simulink model "kinematic_arm_simulation"  (Simulink 7.8)
settings: Solver=FixedStepDiscrete  SolverMode=SingleTasking  StartTime=0.0  StopTime=50  FixedStep=.01  RelTol=1e-3  AbsTol=1e-6
undefined symbols (not defined in the file or in its folder): DiscIntNeverNeededParam, forward_kinematics, inverse_kinematics
libraries: simulink x2
settings Model: Creator=sschaal  LastModifiedBy=okhan  ExtModeAutoUpdateStatusClock=off
settings DataIOCC: LimitDataPoints=off  SaveOutput=off
settings OptimizationCC: BlockReduction=off  BooleanDataType=off  InitFltsAndDblsToZero=on
settings DebuggingCC: SaveWithParameterizedLinksMsg=none  SignalResolutionControl=TryResolveAllWithWarning  SolverPrmCheckMsg=none  MultiTaskDSMMsg=warning  MultiTaskCondExecSysMsg=none  FcnCallInpInsideContextMsg=Use local settings  StrictBusMsg=None
settings HardwareCC: TargetUnknown=on
settings RTWCC: IncludeERTFirstTime=on
settings GRTTargetCC: TargetFcnLib=ansi_tfl_tmw.mat

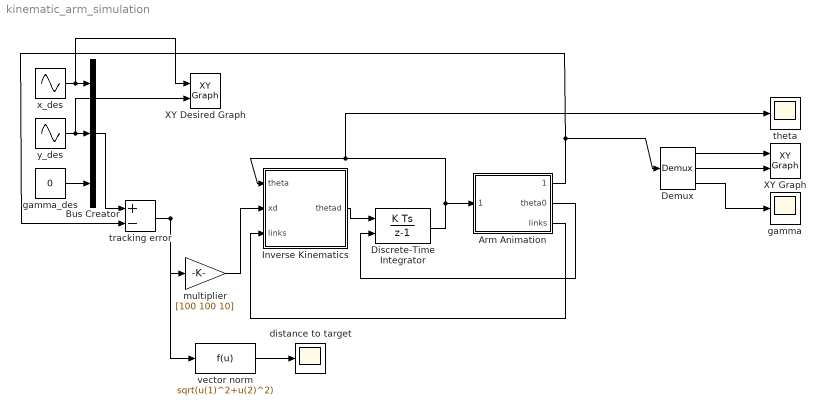
== system kinematic_arm_simulation ==
  Arm Animation : Subsystem  mask(ArmAnimation){links=[0.1 0.0 0.1 0.0 0.1 0.0 0.1 0.0], theta0=[0.0; 0.125; 0.0; 0.125; 0.0; 0.125; 0.0; 0.125], ts=.05}
      mask prompts: links "Link Lengths"; theta0 "Initial Posture"; ts "Sample time:"
  Bus Creator : BusCreator  Inputs=3
  Demux : Demux  Outputs=3
  Discrete-Time Integrator : DiscreteIntegrator  InitialConditionSource=external  SampleTime=0.01  UpperSaturationLimit=[inf .1 inf .1 inf .1 inf .1]  LowerSaturationLimit=[-inf 0 -inf 0 -inf 0 -inf 0]  ICPrevOutput=DiscIntNeverNeededParam  ICPrevScaledInput=DiscIntNeverNeededParam
  Inverse Kinematics : Subsystem
      mask Type: Inverse Kinematics
  XY Desired Graph : simulink/Sinks/XY Graph  xmin=0.2  xmax=1  ymin=-1  ymax=1  st=-1
  XY Graph : simulink/Sinks/XY Graph  xmin=0.2  xmax=1  ymin=-1  ymax=1  st=-1
  distance to target : Scope
      settings: TickLabels=on  TimeRange=50  YMin=0  YMax=0.016  DataFormat=Array
  gamma : Scope
      settings: TimeRange=50  YMin=-3e-15  YMax=5e-15
  gamma_des : Constant  Value=0
  multiplier : Gain  Gain=[100 100 10]  SaturateOnIntegerOverflow=on  OutDataTypeStr=Inherit: Same as input  ParamDataTypeStr=Inherit: Same as input
  theta : Scope
      settings: YMin=-0.8  YMax=0.9  SaveName=ScopeData2
  tracking error : Sum  Inputs=+-  SaturateOnIntegerOverflow=on  InputSameDT=on  OutDataTypeStr=Inherit: Same as first input
  vector norm : Fcn  Expr=sqrt(u(1)^2+u(2)^2)
  x_des : Sin  Amplitude=.3  Bias=.6  Frequency=pi/5  Phase=pi/2  SampleTime=0
  y_des : Sin  Amplitude=.6  Frequency=pi/5  SampleTime=0
  wires:
  multiplier/1 -> Inverse Kinematics/2(xd)
  Inverse Kinematics/1(thetad) -> Discrete-Time Integrator/1
  Discrete-Time Integrator/1 -> Arm Animation/1(Position), Inverse Kinematics/1(theta), theta/1
  Demux/1 -> XY Graph/1
  Demux/2 -> XY Graph/2
  Arm Animation/3(links) -> Inverse Kinematics/3(links)
  Arm Animation/2(theta0) -> Discrete-Time Integrator/2
  Arm Animation/1("[x,y,gamma]") -> tracking error/2, Demux/1
  tracking error/1 -> multiplier/1, vector norm/1
  vector norm/1 -> distance to target/1
  Bus Creator/1 -> tracking error/1
  x_des/1 -> Bus Creator/1, XY Desired Graph/1
  y_des/1 -> Bus Creator/2, XY Desired Graph/2
  gamma_des/1 -> Bus Creator/3
  Demux/3 -> gamma/1

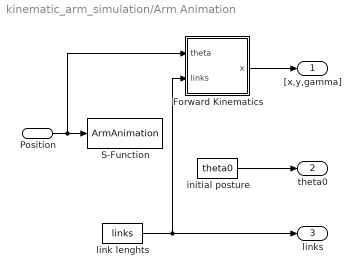
== system kinematic_arm_simulation/Arm Animation ==
  Position : Inport
  Forward Kinematics : Subsystem
      mask Type: Forward Kinematics
  S-Function : S-Function  FunctionName=ArmAnimation  Parameters=ts,theta0,links  EnableBusSupport=off
  initial posture : Constant  Value=theta0
  link lenghts : Constant  Value=links
  "[x,y,gamma]" : Outport
  theta0 : Outport  Port=2
  links : Outport  Port=3
  wires:
  initial posture/1 -> theta0/1
  Position/1 -> S-Function/1, Forward Kinematics/1(theta)
  Forward Kinematics/1(x) -> "[x,y,gamma]"/1
  link lenghts/1 -> links/1, Forward Kinematics/2(links)

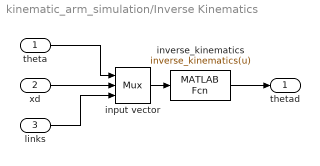
== system kinematic_arm_simulation/Inverse Kinematics ==
  theta : Inport
  xd : Inport  Port=2
  links : Inport  Port=3
  input vector : Mux  Inputs=3
  inverse_kinematics : MATLABFcn  MATLABFcn=inverse_kinematics(u)  OutputDimensions=8
  thetad : Outport  InitialOutput=0
  wires:
  theta/1 -> input vector/1
  xd/1 -> input vector/2
  input vector/1 -> inverse_kinematics/1
  links/1 -> input vector/3
  inverse_kinematics/1 -> thetad/1

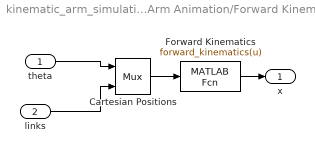
== system kinematic_arm_simulation/Arm Animation/Forward Kinematics ==
  theta : Inport
  links : Inport  Port=2
  Cartesian Positions : Mux  Inputs=2
  Forward Kinematics : MATLABFcn  MATLABFcn=forward_kinematics(u)  OutputDimensions=3
  x : Outport  InitialOutput=0
  wires:
  Forward Kinematics/1 -> x/1
  theta/1 -> Cartesian Positions/1
  links/1 -> Cartesian Positions/2
  Cartesian Positions/1 -> Forward Kinematics/1
